simulink model "PIA_BNO055"  (R2020b)
settings: Solver=VariableStepAuto  StartTime=0.0  StopTime=inf  RelTol=1e-3
model workspace (MAT data in the model file):
  alpha = Simulink.Parameter
  alpha.Value = 0.04
  alpha.DataType = 'auto'
  alpha.Dimensions = [1 1]
  dt = Simulink.Parameter
  dt.Value = 0.01
  dt.DataType = 'auto'
  dt.Dimensions = [1 1]
undefined symbols (not defined in the file or in its folder): serial
libraries: instrumentlib x2
settings Model: EnablePacing=on  Creator=eber_  LastModifiedBy=eber_

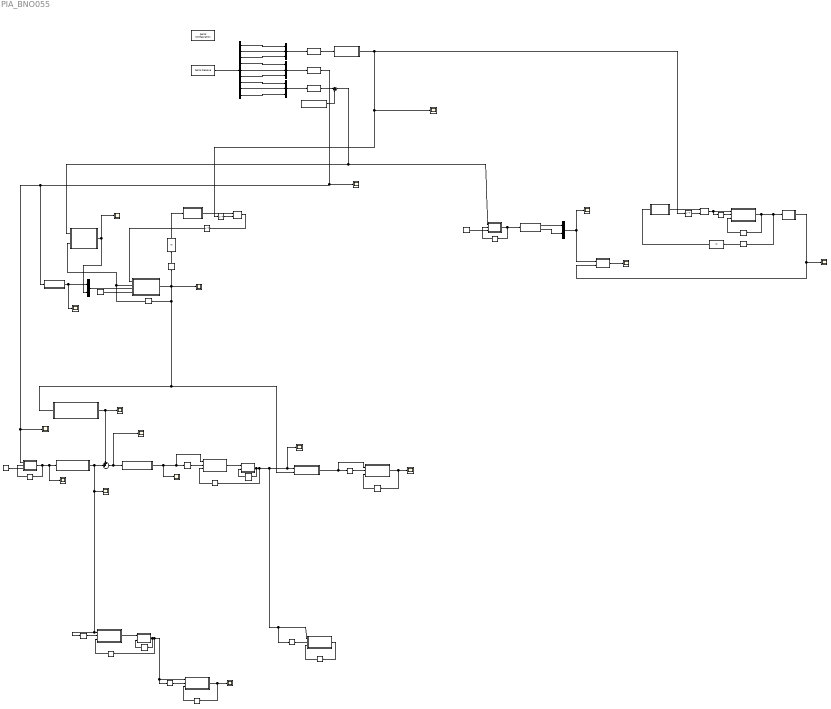
== system PIA_BNO055 ==
  note: Linear Motion
  note: w/ Transformation Matrix
  note: Angles Determination
  note: Average
  note: Data Acquisition and Calibration
  Accelerometer Angles : MATLAB Function  TreatAsAtomicUnit=on
  Axes Change : MATLAB Function  TreatAsAtomicUnit=on
  Axes Transformation : MATLAB Function  TreatAsAtomicUnit=on
  Band Rejection : MATLAB Function  TreatAsAtomicUnit=on
  Chart : Stateflow chart  TreatAsAtomicUnit=on
  Compensation Calculation : MATLAB Function  TreatAsAtomicUnit=on
  Constant : Constant  Value=[-5.2188; 35.3125; 21.1563]
  Data Type Conversion : DataTypeConversion  OutDataTypeStr=double
  Data Type Conversion1 : DataTypeConversion  OutDataTypeStr=double
  Data Type Conversion2 : DataTypeConversion  OutDataTypeStr=double
  Delay1 : Delay  DelayLength=5
  Delay2 : Delay  DelayLength=5
  Demux4 : Demux  Outputs=9
  Displacement : Scope
  Displacement2 : Scope
  IC10 : InitialCondition  Value=[0; 0; 0]
  IC11 : InitialCondition  Value=[0, 0, 0]
  Integration : MATLAB Function  TreatAsAtomicUnit=on
  Integration1 : MATLAB Function  TreatAsAtomicUnit=on
  Integration2 : MATLAB Function  TreatAsAtomicUnit=on
  Integration3 : MATLAB Function  TreatAsAtomicUnit=on
  Integration4 : MATLAB Function  TreatAsAtomicUnit=on
  MATLAB Function13 : MATLAB Function  TreatAsAtomicUnit=on
  MATLAB Function14 : MATLAB Function  TreatAsAtomicUnit=on
  MATLAB Function18 : MATLAB Function  TreatAsAtomicUnit=on
  MATLAB Function20 : MATLAB Function  TreatAsAtomicUnit=on
  MATLAB Function21 : MATLAB Function  TreatAsAtomicUnit=on
  MATLAB Function24 : MATLAB Function  TreatAsAtomicUnit=on
  MATLAB Function25 : MATLAB Function  TreatAsAtomicUnit=on
  Matrix Multiply7 : Product  Multiplication=Matrix(*)
  Matrix Multiply8 : Product  Multiplication=Matrix(*)
  Memory{35..36,38,41,47,50} (6 alike) : Memory  InitialCondition=[0, 0, 0]
  Memory{37,39..40,42..46,48..49,51} (11 alike) : Memory
  Mux16 : Mux  Inputs=3
  Mux17 : Mux  Inputs=2
  Mux18 : Mux  Inputs=2
  Mux3 : Mux  Inputs=3
  Mux4 : Mux  Inputs=3
  Scope{1..3,23..28,30,32,35..37,39} (15 alike) : Scope
  Serial Configuration : instrumentlib/Serial Configuration  Priority=-200000  ComPortMenu=<Please select a port...>  ComPort=COM3  ObjConstructor=serial('COM3');  BaudRate=115200  DataBits=8  Parity=none  StopBits=1  FlowControl=none  Timeout=10  ByteOrder=LittleEndian
  Serial Receive : instrumentlib/Serial Receive  ComPortMenu=<Please select a port...>  ComPort=COM3  ObjConstructor=serial('COM3');  Terminator=<none>  DataSize="[1  9]"  DataType=single  EnableBlockingMode=on  ActionDataUnavailable=Output last received value  CustomValue=0  SampleTime=0.02
  Sum : Sum  Inputs=|+-
  Sum1 : Sum  Inputs=++|
  Tilt compensation : MATLAB Function  TreatAsAtomicUnit=on
  Transformation Matrix : MATLAB Function  TreatAsAtomicUnit=on
  Transformation Matrix7 : MATLAB Function  TreatAsAtomicUnit=on
  Transpose10 : Math  Operator=transpose  SaturateOnIntegerOverflow=on
  Transpose11 : Math  Operator=transpose  SaturateOnIntegerOverflow=on
  Transpose12 : Math  Operator=transpose  SaturateOnIntegerOverflow=on
  Trapezoid8 : MATLAB Function  TreatAsAtomicUnit=on
  Velocity Frame Rotation : MATLAB Function  TreatAsAtomicUnit=on
  alpha10 : Constant  Value=0.055
  alpha7 : Constant  Value=0.04
  alpha8 : Constant  Value=0.5
  wires:
  Data Type Conversion/1 -> Chart/1(gyroIn)
  Serial Receive/1 -> Demux4/1
  Demux4/2 -> Mux3/2
  Demux4/1 -> Mux3/1
  Demux4/3 -> Mux3/3
  Demux4/5 -> Mux4/2
  Demux4/4 -> Mux4/1
  Demux4/6 -> Mux4/3
  Mux3/1 -> Data Type Conversion/1  "gyro"
  Mux4/1 -> Data Type Conversion1/1  "acc"
  Demux4/7 -> Mux16/1
  Demux4/8 -> Mux16/2
  Demux4/9 -> Mux16/3
  Mux16/1 -> Data Type Conversion2/1  "mag"
  Constant/1 -> Sum/2
  Tilt compensation/1(psi) -> Mux17/2, Scope23/1
  Memory35/1 -> Tilt compensation/2(angles), MATLAB Function13/2(Xa)
  MATLAB Function13/1(X) -> Memory48/1, Scope26/1, Memory35/1, Compensation Calculation/1(euler), Velocity Frame Rotation/2(euler)
  alpha7/1 -> MATLAB Function13/4(alpha)
  MATLAB Function14/1(angAcc) -> Mux17/1, Scope39/1
  Mux17/1 -> MATLAB Function13/3(angAcc)
  Compensation Calculation/1(gravB) -> Scope24/1, Sum1/1
  Band Rejection/1(bandRejected) -> Scope25/1, Memory37/1, Integration/1(X_dot)  "raw"
  Memory36/1 -> Integration/3(X)
  Memory37/1 -> Integration/2(X_dot_prev)
  Integration/1(X_out) -> MATLAB Function20/1(u)
  Delay2/1 -> MATLAB Function20/2(uA)
  Integration1/1(X_out) -> Displacement/1, Memory38/1
  Memory39/1 -> Integration1/2(X_dot_prev)
  Memory38/1 -> Integration1/3(X)
  Velocity Frame Rotation/1(velInertial) -> Integration1/1(X_dot), Memory39/1  "raw"
  Sum/1 -> Tilt compensation/1(mag), MATLAB Function24/1(U)
  Memory42/1 -> MATLAB Function24/2(Xa)
  MATLAB Function24/1(X) -> Accelerometer Angles/1(acc), Memory42/1
  alpha10/1 -> MATLAB Function24/3(alpha)
  Transformation Matrix7/1(H) -> Matrix Multiply7/1
  Memory45/1 -> IC10/1
  IC10/1 -> Transformation Matrix7/1(Phi)
  Matrix Multiply7/1 -> Trapezoid8/1(Euler_dot), Memory44/1
  Transpose10/1 -> Matrix Multiply7/2
  Trapezoid8/1(Euler_out) -> Memory43/1, Axes Change/1(u), Memory45/1
  Memory44/1 -> Trapezoid8/2(Euler_dot_prev)
  Memory43/1 -> Trapezoid8/3(Euler)
  Accelerometer Angles/1(phi_acc) -> Mux18/1
  Accelerometer Angles/2(theta_acc) -> Mux18/2
  Mux18/1 -> MATLAB Function25/1(acc), Scope37/1
  Axes Change/1(y) -> Scope36/1, MATLAB Function25/2(gyro)
  MATLAB Function25/1(prom) -> Scope35/1
  Memory48/1 -> IC11/1
  IC11/1 -> Transformation Matrix/1(Phi)
  Chart/1(gyroOut) -> Transpose10/1, Scope3/1, Transpose11/1
  Matrix Multiply8/1 -> Transpose12/1
  Transpose11/1 -> Matrix Multiply8/2
  Transformation Matrix/1(H) -> Matrix Multiply8/1
  Transpose12/1 -> MATLAB Function13/1(G)
  Sum1/1 -> Band Rejection/1(compensatedAcc), Scope32/1
  alpha8/1 -> MATLAB Function18/3(alpha)
  Memory40/1 -> MATLAB Function18/2(Xa)
  MATLAB Function18/1(X) -> Memory40/1, Axes Transformation/1(accNWUbody), Scope30/1
  MATLAB Function20/1(y) -> Delay2/1, Memory36/1, Scope1/1, Velocity Frame Rotation/1(velBody), Integration2/1(X_dot), Memory46/1  "raw"
  Memory41/1 -> Integration2/3(X)
  Memory46/1 -> Integration2/2(X_dot_prev)
  Integration2/1(X_out) -> Memory41/1
  Delay1/1 -> MATLAB Function21/2(uA)
  Integration4/1(X_out) -> MATLAB Function21/1(u)
  Memory49/1 -> Integration4/2(X_dot_prev)
  Memory47/1 -> Integration4/3(X)
  Axes Transformation/1(accNEDbody) -> Sum1/2, Integration4/1(X_dot), Memory49/1, Scope28/1  "raw"
  Integration3/1(X_out) -> Displacement2/1, Memory50/1
  Memory51/1 -> Integration3/2(X_dot_prev)
  Memory50/1 -> Integration3/3(X)
  MATLAB Function21/1(y) -> Memory47/1, Integration3/1(X_dot), Memory51/1, Delay1/1  "raw"
  Data Type Conversion1/1 -> MATLAB Function14/1(acc), Scope27/1, MATLAB Function18/1(U), Scope2/1
  Data Type Conversion2/1 -> Sum/1

== matlab function PIA_BNO055/MATLAB Function14 ==
  data: acc input; angAcc output
function angAcc  = fcn(acc)
ax = acc(1);
ay = acc(2);
az = acc(3);

phi_acc = atand(ay/sqrt(ax^2 + az^2));
theta_acc = atand(ax/sqrt(ay^2 + az^2));


angAcc = [phi_acc, theta_acc]

== matlab function PIA_BNO055/Compensation Calculation ==
  data: euler input; gravB output
function gravB = fcn(euler)
euler = deg2rad(euler);
phi = euler(1);
theta = euler(2);
psi = euler(3);
R = eul2rotm([psi, theta, phi]);
gravI = [0; 0; 9.45];
gravB = R'*gravI;

== matlab function PIA_BNO055/Axes Transformation ==
  data: accNWUbody input; accNEDbody output
function accNEDbody = fcn(accNWUbody)
accNEDbody = [accNWUbody(1); -accNWUbody(2); -accNWUbody(3)];

== matlab function PIA_BNO055/Integration ==
  data: X_dot input; X_dot_prev input; X_out output; X input
function X_out = fcn(X_dot, X_dot_prev, X)
dt = 0.02;

phi_dot = X_dot(1);
theta_dot = X_dot(2);
psi_dot = X_dot(3);


phi_dot_prev = X_dot_prev(1);
theta_dot_prev = X_dot_prev(2);
psi_dot_prev = X_dot_prev(3);


phi = X(1);
theta = X(2);
psi = X(3);


phi = phi + dt*phi_dot - dt*((phi_dot - phi_dot_prev)/2);
theta = theta + dt*theta_dot - dt*((theta_dot - theta_dot_prev)/2);
psi = psi + dt*psi_dot - dt*((psi_dot - psi_dot_prev)/2);

X_out = [phi; theta; psi];

== matlab function PIA_BNO055/Band Rejection ==
  data: compensatedAcc input; bandRejected output
function bandRejected = fcn(compensatedAcc)
x = compensatedAcc(1);
y = compensatedAcc(2);
z = compensatedAcc(3);

if abs(x) < 0.1
    x = 0;
end

if abs(y) < 0.1
    y = 0;
end

if abs(z) < 0.1
    z = 0;
end

bandRejected = [x, y, z];

== matlab function PIA_BNO055/Velocity Frame Rotation ==
  data: velBody input; velInertial output; euler input
function velInertial = fcn(velBody, euler)
euler = deg2rad(euler);
phi = euler(1);
theta = euler(2);
psi = euler(3);
R = eul2rotm([psi, theta, phi]);
velInertial = R*velBody;

== matlab function PIA_BNO055/MATLAB Function20 ==
  data: u input; y output; uA input
function y = fcn(u, uA)

if u == uA
    y = [0; 0; 0];
else
    y = u;
end

== matlab function PIA_BNO055/MATLAB Function18 ==
  data: U input; X output; Xa input; alpha input
function X = fcn(U, Xa, alpha)
X = alpha*U + (1 - alpha)*Xa;

== matlab function PIA_BNO055/Accelerometer Angles ==
  data: acc input; phi_acc output; theta_acc output
function [phi_acc, theta_acc] = fcn(acc)
ax = acc(1);
ay = acc(2);
az = acc(3);

phi_acc = atand(ay/sqrt(ax^2 + az^2));
theta_acc = atand(ax/sqrt(ay^2 + az^2));

== matlab function PIA_BNO055/MATLAB Function24 ==
  data: U input; X output; Xa input; alpha input
function X = fcn(U, Xa, alpha)
X = alpha*U + (1 - alpha)*Xa;

== matlab function PIA_BNO055/Transformation Matrix7 ==
  data: Phi input; H output
function H = fcn(Phi)
Phi = deg2rad(Phi);

phi = Phi(1);
theta = Phi(2);
psi = Phi(3);

H = [1 tan(theta)*sin(phi) tan(theta)*cos(phi);
    0 cos(phi) -sin(phi);
    0 sin(phi)/cos(theta) cos(phi)/cos(theta)];

== matlab function PIA_BNO055/Trapezoid8 ==
  data: Euler_dot input; Euler_dot_prev input; Euler_out output; Euler input
function Euler_out = fcn(Euler_dot, Euler_dot_prev, Euler)
dt = 0.02;

phi_dot = Euler_dot(1);
theta_dot = Euler_dot(2);
psi_dot = Euler_dot(3);


phi_dot_prev = Euler_dot_prev(1);
theta_dot_prev = Euler_dot_prev(2);
psi_dot_prev = Euler_dot_prev(3);


phi = Euler(1);
theta = Euler(2);
psi = Euler(3);


phi = phi + dt*phi_dot - dt*((phi_dot - phi_dot_prev)/2);
theta = theta + dt*theta_dot - dt*((theta_dot - theta_dot_prev)/2);
psi = psi + dt*psi_dot - dt*((psi_dot - psi_dot_prev)/2);

Euler_out = [phi; theta; psi];

== matlab function PIA_BNO055/MATLAB Function25 ==
  data: acc input; prom output; gyro input
function prom = fcn(acc, gyro)
phiprom = (acc(1) + gyro(1))/2;
thetaprom = (acc(2) + gyro(2))/2;
prom = [phiprom, thetaprom];

== matlab function PIA_BNO055/Axes Change ==
  data: u input; y output
function y = fcn(u)
phi = u(1);
theta = -u(2);
psi = -u(3);

y = [phi, theta, psi]

== matlab function PIA_BNO055/Transformation Matrix ==
  data: Phi input; H output
function H = fcn(Phi)
Phi = deg2rad(Phi);

phi = Phi(1);
theta = Phi(2);
psi = Phi(3);

H = [1 tan(theta)*sin(phi) tan(theta)*cos(phi);
    0 cos(phi) -sin(phi);
    0 sin(phi)/cos(theta) cos(phi)/cos(theta)];

== matlab function PIA_BNO055/MATLAB Function21 ==
  data: u input; y output; uA input
function y = fcn(u, uA)

if u == uA
    y = [0; 0; 0];
else
    y = u;
end

== matlab function PIA_BNO055/Integration1 ==
  data: X_dot input; X_dot_prev input; X_out output; X input
function X_out = fcn(X_dot, X_dot_prev, X)
dt = 0.02;

phi_dot = X_dot(1);
theta_dot = X_dot(2);
psi_dot = X_dot(3);


phi_dot_prev = X_dot_prev(1);
theta_dot_prev = X_dot_prev(2);
psi_dot_prev = X_dot_prev(3);


phi = X(1);
theta = X(2);
psi = X(3);


phi = phi + dt*phi_dot - dt*((phi_dot - phi_dot_prev)/2);
theta = theta + dt*theta_dot - dt*((theta_dot - theta_dot_prev)/2);
psi = psi + dt*psi_dot - dt*((psi_dot - psi_dot_prev)/2);

X_out = [phi; theta; psi];

== matlab function PIA_BNO055/Integration2 ==
  data: X_dot input; X_dot_prev input; X_out output; X input
function X_out = fcn(X_dot, X_dot_prev, X)
dt = 0.02;

phi_dot = X_dot(1);
theta_dot = X_dot(2);
psi_dot = X_dot(3);


phi_dot_prev = X_dot_prev(1);
theta_dot_prev = X_dot_prev(2);
psi_dot_prev = X_dot_prev(3);


phi = X(1);
theta = X(2);
psi = X(3);


phi = phi + dt*phi_dot - dt*((phi_dot - phi_dot_prev)/2);
theta = theta + dt*theta_dot - dt*((theta_dot - theta_dot_prev)/2);
psi = psi + dt*psi_dot - dt*((psi_dot - psi_dot_prev)/2);

X_out = [phi; theta; psi];

== matlab function PIA_BNO055/Integration3 ==
  data: X_dot input; X_dot_prev input; X_out output; X input
function X_out = fcn(X_dot, X_dot_prev, X)
dt = 0.02;

phi_dot = X_dot(1);
theta_dot = X_dot(2);
psi_dot = X_dot(3);


phi_dot_prev = X_dot_prev(1);
theta_dot_prev = X_dot_prev(2);
psi_dot_prev = X_dot_prev(3);


phi = X(1);
theta = X(2);
psi = X(3);


phi = phi + dt*phi_dot - dt*((phi_dot - phi_dot_prev)/2);
theta = theta + dt*theta_dot - dt*((theta_dot - theta_dot_prev)/2);
psi = psi + dt*psi_dot - dt*((psi_dot - psi_dot_prev)/2);

X_out = [phi; theta; psi];

== matlab function PIA_BNO055/Integration4 ==
  data: X_dot input; X_dot_prev input; X_out output; X input
function X_out = fcn(X_dot, X_dot_prev, X)
dt = 0.02;

phi_dot = X_dot(1);
theta_dot = X_dot(2);
psi_dot = X_dot(3);


phi_dot_prev = X_dot_prev(1);
theta_dot_prev = X_dot_prev(2);
psi_dot_prev = X_dot_prev(3);


phi = X(1);
theta = X(2);
psi = X(3);


phi = phi + dt*phi_dot - dt*((phi_dot - phi_dot_prev)/2);
theta = theta + dt*theta_dot - dt*((theta_dot - theta_dot_prev)/2);
psi = psi + dt*psi_dot - dt*((psi_dot - psi_dot_prev)/2);

X_out = [phi; theta; psi];

== stateflow chart PIA_BNO055/Chart ==
  state initialSample
    entry:
    gyroOut = [0, 0, 0];
    pSum = 0;
    qSum = 0;
    rSum = 0;
    counter = 0;
    during:
    p = gyroIn(1);
    q = gyroIn(2);
    r = gyroIn(3);
    counter = counter + 1;
    pSum = pSum + p;
    qSum = qSum + q;
    rSum = rSum + r;
  state average
    entry:
    pOffset = pSum/counter;
    qOffset = qSum/counter;
    rOffset = rSum/counter;
    exit:
    offsets = [pOffset; qOffset; rOffset];
  state dataAcquisition
    during:
    p = gyroIn(1);
    q = gyroIn(2);
    r = gyroIn(3);
    pcorr = p - pOffset;
    qcorr = q - qOffset;
    rcorr = r - rOffset;
    gyroOut = [pcorr, qcorr, rcorr];
  (default) -> initialSample
  initialSample -> average : after(10, sec)
  average -> dataAcquisition
  data: counter local; p local; pOffset local; pSum local; r local; rOffset local; rSum local; q local; qOffset local; qSum local; offsets local; gyroOut output; pcorr local; qcorr local; rcorr local; gyroIn input

== matlab function PIA_BNO055/Tilt compensation ==
  data: mag input; psi output; angles input
function psi = fcn(mag, angles)
X = mag(1);
Y = mag(2);
Z = mag(3);
phi = angles(1);
theta = -angles(2);
Xh = X*cosd(theta) + Y*sind(theta)*sind(phi) + Z*cosd(phi)*sind(theta);
Yh = Y*cosd(phi) - Z*sind(phi);

psi = atan2d(Yh,Xh);


% Xh = X*cos(theta) + Y*sin(theta)*sin(phi) + Z*cos(phi)*sin(theta);
% Yh = Y*cos(phi) - Z*sin(phi);

% eul = [0 theta phi];
% rotmZYX = eul2rotm(eul)
% body = [X; Y; Z];
% inertial = rotmZYX*body;
% Xh = inertial(1);
% Yh = inertial(2);
% Zh = inertial(3);

== matlab function PIA_BNO055/MATLAB Function13 ==
  data: G input size=[1 3]; X output size=[1 3]; Xa input size=[1 3]; angAcc input size=[1 3]; alpha input
function X = fcn(G, Xa, angAcc, alpha)
dt = 0.02;
G = [G(1), -G(2), -G(3)];
X = (1 - alpha)*(Xa + G*dt) + alpha*angAcc;
